simulink model "LMS_cs_old"  (R2023a)
settings: Solver=ode5  StartTime=0.0  StopTime=inf  FixedStep=1/200  RelTol=1e-3
PreLoadFcn:
  | mbxruntime.callbacks.PreLoadFcn(bdroot);
PostLoadFcn:
  | mbxruntime.callbacks.PostLoadFcn(bdroot);
InitFcn:
  | mbxruntime.callbacks.InitFcn(bdroot);
StartFcn:
  | mbxruntime.callbacks.StartFcn(bdroot);
StopFcn:
  | mbxruntime.callbacks.StopFcn(bdroot);
model workspace (MAT data in the model file):
  mbox_table : object (value not decoded)
  model_closed = 0
  sim_status = 0
undefined symbols (not defined in the file or in its folder): DiscIntNeverNeededParam, WheelL0, WheelL1, WheelR0, WheelR1
libraries: simulink x462, simulink_extras x117, PreScanSimulinkLibrary x33, PreScanUsefulBlocks x6, instrumentseriallib x5, simulink_need_slupdate x1
(part 41 of 68)

== system LMS_cs_old/BMW_X5_SUV_8/Dynamics_Simple_3D/Chassis/Bicycle_model_[XYZ] ==
  DeltaWheel_[rad] : Inport
  BrakePressure_[bar] : Inport  Port=2
  DriveTorque_[Nm] : Inport  Port=3
  v0_[ms-1] : Inport  Port=4
  |vx|_[ms-1] : Inport  Port=5
  Fy_rear_[N] : Inport  Port=6
  Fy_front_[N] : Inport  Port=7
  TyreInfo_in : Inport  Port=8
  Bus Creator : BusCreator  Inputs=4
  Fyi --> Fy / Mz : Subsystem
  Goto Tag Visibility2 : GotoTagVisibility  GotoTag=penetrationfrontleft
  Goto Tag Visibility3 : GotoTagVisibility  GotoTag=penetrationfrontright
  Goto Tag Visibility4 : GotoTagVisibility  GotoTag=penetrationrearright
  Goto Tag Visibility5 : GotoTagVisibility  GotoTag=penetrationrearleft
  RoadContact : Subsystem
  Terminator : Terminator
  X_Motion : Subsystem
  Y & Yaw_Motion : Subsystem
  "Z, Pitch_Motion & Roll_Motion" : Subsystem
  Z_Motion unsprung mass : Subsystem
  |vx|_[ms-1]1 : Outport
  vy_[ms-1] : Outport  Port=2
  vz_[ms-1] : Outport  Port=3
  RollAngle_[rad] : Outport  Port=4
  RollRate_[rads-1] : Outport  Port=5
  YawAngle_[rads-1] : Outport  Port=6
  Vx_[ms-1] : Outport  Port=7
  PitchAngle_[rad] : Outport  Port=8
  YawAngle_[rad] : Outport  Port=9
  ax_[ms-2] : Outport  Port=10
  ay_[ms-2] : Outport  Port=11
  z_wheel_[m] : Outport  Port=12
  tag scope: penetrationfrontleft=scoped, penetrationfrontright=scoped, penetrationrearleft=scoped, penetrationrearright=scoped
  wires:
  TyreInfo_in/1 -> RoadContact/1(TyreInfo_in)
  Bus Creator/1 -> z_wheel_[m]/1
  "Z, Pitch_Motion & Roll_Motion"/2(vz_[ms-1]) -> vz_[ms-1]/1  "vz_[ms-1]"
  v0_[ms-1]/1 -> X_Motion/3(v0_[ms-1])  "v0_[ms-1]"
  [slope] -> X_Motion/4(slope_[rad])
  RoadContact/4(depth_RR [m]) -> [penetrationrearright]
  RoadContact/3(depth_RL [m]) -> [penetrationrearleft]
  RoadContact/2(depth_FR [m]) -> [penetrationfrontright]
  RoadContact/1(depth_FL [m]) -> [penetrationfrontleft]
  Y & Yaw_Motion/5(YawAngle_[rad]) -> YawAngle_[rad]/1  "YawAngle_[rad]"
  [az] -> Z_Motion unsprung mass/2(az_[ms-2])
  [FdampRR] -> Z_Motion unsprung mass/10(FdampRR_[N])
  [FdampRL] -> Z_Motion unsprung mass/9(FdampRL_[N])
  [FspringRR] -> Z_Motion unsprung mass/8(FspringRR_[N])
  [FspringRL] -> Z_Motion unsprung mass/7(FspringRL_[N])
  [FdampFR] -> Z_Motion unsprung mass/6(FdampFR_[N])
  [FdampFL] -> Z_Motion unsprung mass/5(FdampFL_[N])
  [FspringFR] -> Z_Motion unsprung mass/4(FspringFR_[N])
  [FspringFL] -> Z_Motion unsprung mass/3(FspringFL_[N])
  [pitch] -> Z_Motion unsprung mass/1(pitch_[rad])
  Z_Motion unsprung mass/4(z_wheelRR_[m]) -> Bus Creator/4, [z_wheelRR]  "z_wheelRR_[m]"
  Z_Motion unsprung mass/3(z_wheelRL_[m]) -> Bus Creator/3, [z_wheelRL]  "z_wheelRL_[m]"
  Z_Motion unsprung mass/2(z_wheelFR_[m]) -> Bus Creator/2, [z_wheelFR]  "z_wheelFR_[m]"
  Z_Motion unsprung mass/1(z_wheelFL_[m]) -> Bus Creator/1, [z_wheelFL]  "z_wheelFL_[m]"
  [z_wheelRR] -> "Z, Pitch_Motion & Roll_Motion"/9(z_wheelRR_[m])
  [z_wheelRL] -> "Z, Pitch_Motion & Roll_Motion"/8(z_wheelRL_[m])
  [z_wheelFR] -> "Z, Pitch_Motion & Roll_Motion"/7(z_wheelFR_[m])
  [z_wheelFL] -> "Z, Pitch_Motion & Roll_Motion"/6(z_wheelFL_[m])
  [pitch] -> "Z, Pitch_Motion & Roll_Motion"/1(pitch_[rad])
  "Z, Pitch_Motion & Roll_Motion"/13(FdampRR_[N]) -> [FdampRR]
  "Z, Pitch_Motion & Roll_Motion"/12(FdampRL_[N]) -> [FdampRL]
  "Z, Pitch_Motion & Roll_Motion"/11(FspringRR_[N]) -> [FspringRR]
  "Z, Pitch_Motion & Roll_Motion"/10(FspringRL_[N]) -> [FspringRL]
  "Z, Pitch_Motion & Roll_Motion"/9(FdampFR_[N]) -> [FdampFR]
  "Z, Pitch_Motion & Roll_Motion"/8(FdampFL_[N]) -> [FdampFL]
  "Z, Pitch_Motion & Roll_Motion"/7(FspringFR_[N]) -> [FspringFR]
  "Z, Pitch_Motion & Roll_Motion"/6(FspringFL_[N]) -> [FspringFL]
  "Z, Pitch_Motion & Roll_Motion"/5(RollRate_[rads-1]) -> RollRate_[rads-1]/1
  "Z, Pitch_Motion & Roll_Motion"/3(az_[ms-2]) -> [az]
  [dYaw] -> X_Motion/6(dYaw_[rads-1])
  [vy] -> X_Motion/5(vy_[ms-1])
  Fyi --> Fy / Mz/1(Fy_[N]) -> Y & Yaw_Motion/2(Fy_[N])  "Fy_[N]"
  Fyi --> Fy / Mz/2(Mz_[Nm]) -> Y & Yaw_Motion/3(Mz_[Nm])  "Mz_[Nm]"
  Y & Yaw_Motion/1(|vx|_[ms-1]1) -> |vx|_[ms-1]1/1  "|vx|_[ms-1]"
  Y & Yaw_Motion/2(vy_[ms-1]) -> [vy], vy_[ms-1]/1  "vy_[ms-1]"
  BrakePressure_[bar]/1 -> X_Motion/2(BrakePressure_[bar])  "BrakePressure_[bar]"
  DriveTorque_[Nm]/1 -> X_Motion/1(DriveTorque_[Nm])  "DriveTorque_[Nm]"
  X_Motion/2(ax_[ms-2]) -> ax_[ms-2]/1, [ax]  "ax_[ms-2]"
  X_Motion/1(vx_[ms-1]) -> Vx_[ms-1]/1, [vx]  "vx_[ms-1]"
  [ax] -> "Z, Pitch_Motion & Roll_Motion"/4(ax)
  DeltaWheel_[rad]/1 -> Fyi --> Fy / Mz/1(DeltaWheel_[rad])
  Fy_front_[N]/1 -> Fyi --> Fy / Mz/2(Fy_f_[N])
  Fy_rear_[N]/1 -> Fyi --> Fy / Mz/3(Fy_r_[N])
  |vx|_[ms-1]/1 -> Y & Yaw_Motion/1(|vx|_[ms-1])
  Y & Yaw_Motion/3(ay_[ms-2]) -> [ay], ay_[ms-2]/1
  [ay] -> "Z, Pitch_Motion & Roll_Motion"/5(ay)
  "Z, Pitch_Motion & Roll_Motion"/4(RollAngle_[rad]) -> RollAngle_[rad]/1
  [dYaw] -> "Z, Pitch_Motion & Roll_Motion"/3(dYaw)
  [vx] -> "Z, Pitch_Motion & Roll_Motion"/2(vx)
  Y & Yaw_Motion/4(dYawAngle_[rads-1]) -> YawAngle_[rads-1]/1, [dYaw]  "dYawAngle_[rads-1]"
  "Z, Pitch_Motion & Roll_Motion"/1(pitchAngle_[rad]) -> [pitch], PitchAngle_[rad]/1  "PitchAngle_[rad]"
  RoadContact/5(z) -> Terminator/1
  RoadContact/6(slope) -> [slope]
  RoadContact/7(banking) -> [banking]
  [banking] -> "Z, Pitch_Motion & Roll_Motion"/10(banking)

== system LMS_cs_old/BMW_X5_SUV_8/Dynamics_Simple_3D/Chassis/FrontTyre ==
  note: relax_on
      | ON: 1
      | OFF: 0
  note: MOTORCYCLE ONLY
  note: VEHICLE + MOTORCYCLE
  note: alpha limiter
      | [-1 ... 1]
  DeltaWheel_[rad] : Inport
  |vx|_[ms-1] : Inport  Port=2
  vy_[ms-1] : Inport  Port=3
  dYawAngle_[rads-1] : Inport  Port=4
  RollAngle_[rad] : Inport  Port=5
  AlphaFront : Subsystem
  Compare To Zero : simulink/Logic and Bit Operations/Compare To Zero  relop===  OutDataTypeStr=boolean  ZeroCross=off
  Configurable Subsystem : Subsystem  BlockChoice=Integrator  mask{ComputationMode=ComputationMode}
      mask prompts: ComputationMode "Computation mode:"
      mask init:
      | SetComputationMode(gcb,ComputationMode);
      settings: AttributesFormatString=%<BlockChoice>  OpenFcn=BringToFront(gcb);  MemberBlocks=Discrete-Time Integrator,Integrator
      settings: TemplateBlock=|
      | PreScanSimulinkLibrary/Configurable Subsystems/integral with reset and limits
      | for slip angle/Configurable
      | Subsystem
  Configurable Subsystem1 : Subsystem  BlockChoice=Integrator  mask{ComputationMode=ComputationMode}
      mask prompts: ComputationMode "Computation mode:"
      mask init:
      | SetComputationMode(gcb,ComputationMode);
      settings: AttributesFormatString=%<BlockChoice>  OpenFcn=BringToFront(gcb);  MemberBlocks=Discrete-Time Integrator,Integrator
      settings: TemplateBlock=|
      | PreScanSimulinkLibrary/Configurable Subsystems/integral with reset/Configurable
      | Subsystem
  Constant : Constant  Value=p.relax_on
  Constant1 : Constant  Value=p.relax_on
  Constant2 : Constant  Value=p.VehMCSwitch
  Data Type Conversion : DataTypeConversion  OutDataTypeStr=double  SaturateOnIntegerOverflow=off  RndMeth=Floor
  If MC : simulink/Logic and Bit Operations/Compare To Constant  relop===  const=2  OutDataTypeStr=uint8  ZeroCross=off
  K_gamma_front : Gain  Gain=p.Kgfront
  Linl : Fcn  Expr=(u(4) - u(5))/p.sigma_front*u(1)
  Linl1 : Fcn  Expr=(u(4) - u(5))/p.sigma_front*u(1)
  Mux1 : Mux  Inputs=3
  Mux2 : Mux  Inputs={3,1,1}
  Mux3 : Mux  Inputs={3,1,1}
  Product : Product  RndMeth=Zero
  Sum : Sum  Inputs=|++  InputSameDT=on  SaturateOnIntegerOverflow=on  OutDataTypeStr=Inherit: Same as first input
  Sum1 : Sum  Inputs=|++
  Switch : Switch  Threshold=0.5
  Switch1 : Switch  Threshold=0.5
  alg.loop : Memory
  due to sign convention : Gain  Gain=-1  SaturateOnIntegerOverflow=on  OutDataTypeStr=Inherit: Same as input  ParamDataTypeStr=Inherit: Same as input
  front_tyre : Gain  Gain=p.Kfront
  FyFront_[N] : Outport
  wires:
  Sum/1 -> Mux2/2, Switch/3  "AlphaStatFront_[rad]"
  Switch/1 -> front_tyre/1  "AlphaFront_[rad]"
  Constant/1 -> Switch/2
  Sum1/1 -> FyFront_[N]/1  "FyFront_[N]"
  Mux2/1 -> Linl/1
  Linl/1 -> Configurable Subsystem/1(In1)
  Configurable Subsystem/1(Out1) -> Mux2/3, Switch/1  "AlphaRelaxFront_[rad]"
  AlphaFront/1(Alpha) -> Sum/1
  Mux1/1 -> AlphaFront/1(In), Mux2/1, Mux3/1
  |vx|_[ms-1]/1 -> Mux1/1, Compare To Zero/1
  vy_[ms-1]/1 -> Mux1/2
  dYawAngle_[rads-1]/1 -> Mux1/3
  alg.loop/1 -> Switch1/3
  Configurable Subsystem1/1(Out1) -> Mux3/3, Switch1/1  "GammaRelaxFront_[rad]"
  Linl1/1 -> Configurable Subsystem1/1(In1)
  Mux3/1 -> Linl1/1
  Constant1/1 -> Switch1/2
  due to sign convention/1 -> alg.loop/1, Mux3/2  "GammaStatFront_[rad]"
  RollAngle_[rad]/1 -> due to sign convention/1
  front_tyre/1 -> Sum1/1
  Constant2/1 -> If MC/1
  If MC/1 -> Data Type Conversion/1
  K_gamma_front/1 -> Product/1
  Product/1 -> Sum1/2
  Data Type Conversion/1 -> Product/2
  Compare To Zero/1 -> [reset]
  [reset] -> Configurable Subsystem/2(In2)
  [reset] -> Configurable Subsystem1/2(In2)
  DeltaWheel_[rad]/1 -> Sum/2  "DeltaWheel_[rad]"
  Switch1/1 -> K_gamma_front/1  "GammaFront_[rad]"

== system LMS_cs_old/BMW_X5_SUV_8/Dynamics_Simple_3D/Chassis/Power Assisted Steering ==
  note: MOTORCYCLE
  note: VEHICLE
  note: Reverse steering direction for negative velocities
  Vx_[ms-1] : Inport
  Delta_in_[deg] : Inport  Port=2
  Constant : Constant
  Constant1 : Constant  Value=p.VehMCSwitch
  Lookup Table : Lookup  InputValues=[0 35 45 100]  Table=[1 1 0.2 0.2]  SaturateOnIntegerOverflow=off
  Multiport Switch : MultiPortSwitch  Inputs=2  SaturateOnIntegerOverflow=off  InputSameDT=off
  Product : Product  Inputs=3  RndMeth=Zero
  Sign : Signum
  Delta_out_[deg] : Outport
  wires:
  Vx_[ms-1]/1 -> Lookup Table/1, Sign/1
  Delta_in_[deg]/1 -> Product/3
  Constant1/1 -> Multiport Switch/1
  Constant/1 -> Multiport Switch/3
  Lookup Table/1 -> Multiport Switch/2
  Multiport Switch/1 -> Product/2
  Product/1 -> Delta_out_[deg]/1
  Sign/1 -> Product/1

== system LMS_cs_old/BMW_X5_SUV_8/Dynamics_Simple_3D/Chassis/RearTyre ==
  note: relax_on
      | ON: 1
      | OFF: 0
  note: MOTORCYCLE ONLY
  note: VEHICLE + MOTORCYCLE
  note: alpha limiter
      | [-1 ... 1]
  |vx|_[ms-1] : Inport
  vy_[ms-1] : Inport  Port=2
  dpsi_[rads-1] : Inport  Port=3
  RollAngle_[rad] : Inport  Port=4
  AlphaRear : Subsystem
  Compare To Zero : simulink/Logic and Bit Operations/Compare To Zero  relop===  OutDataTypeStr=boolean  ZeroCross=off
  Configurable Subsystem : Subsystem  BlockChoice=Integrator  mask{ComputationMode=ComputationMode}
      mask prompts: ComputationMode "Computation mode:"
      mask init:
      | SetComputationMode(gcb,ComputationMode);
      settings: AttributesFormatString=%<BlockChoice>  OpenFcn=BringToFront(gcb);  MemberBlocks=Discrete-Time Integrator,Integrator
      settings: TemplateBlock=|
      | PreScanSimulinkLibrary/Configurable Subsystems/integral with reset and limits
      | for slip angle/Configurable
      | Subsystem
  Configurable Subsystem1 : Subsystem  BlockChoice=Integrator  mask{ComputationMode=ComputationMode}
      mask prompts: ComputationMode "Computation mode:"
      mask init:
      | SetComputationMode(gcb,ComputationMode);
      settings: AttributesFormatString=%<BlockChoice>  OpenFcn=BringToFront(gcb);  MemberBlocks=Discrete-Time Integrator,Integrator
      settings: TemplateBlock=|
      | PreScanSimulinkLibrary/Configurable Subsystems/integral with reset/Configurable
      | Subsystem
  Constant1 : Constant  Value=p.relax_on
  Constant2 : Constant  Value=p.relax_on
  Constant3 : Constant  Value=p.VehMCSwitch
  Data Type Conversion : DataTypeConversion  OutDataTypeStr=double  SaturateOnIntegerOverflow=off  RndMeth=Floor
  If MC : simulink/Logic and Bit Operations/Compare To Constant  relop===  const=2  OutDataTypeStr=uint8  ZeroCross=off
  K_gamma_rear : Gain  Gain=p.Kgrear
  Linl : Fcn  Expr=(u(4) - u(5))/p.sigma_rear*u(1)
  Linl1 : Fcn  Expr=(u(4) - u(5))/p.sigma_rear*u(1)
  Mux1 : Mux  Inputs=3
  Mux2 : Mux  Inputs={3,1,1}
  Mux3 : Mux  Inputs={3,1,1}
  Product : Product  RndMeth=Zero
  Sum1 : Sum  Inputs=|++
  Switch1 : Switch  Threshold=0.5
  Switch2 : Switch  Threshold=0.5
  alg.loop : Memory
  due to sign convention : Gain  Gain=-1  SaturateOnIntegerOverflow=on  OutDataTypeStr=Inherit: Same as input  ParamDataTypeStr=Inherit: Same as input
  rear_tyre : Gain  Gain=p.Krear
  FyRear_[N] : Outport
  wires:
  AlphaRear/1(Alpha) -> Switch1/3, Mux2/2  "AlphaStatRear_[rad]"
  Switch1/1 -> rear_tyre/1  "AlphaRear_[rad]"
  Constant1/1 -> Switch1/2
  Sum1/1 -> FyRear_[N]/1  "FyRear_[N]"
  Mux2/1 -> Linl/1
  Linl/1 -> Configurable Subsystem/1(In1)
  Configurable Subsystem/1(Out1) -> Mux2/3, Switch1/1  "AlphaRelaxRear_[rad]"
  Mux1/1 -> AlphaRear/1(In), Mux2/1, Mux3/1
  |vx|_[ms-1]/1 -> Mux1/1, Compare To Zero/1
  vy_[ms-1]/1 -> Mux1/2
  dpsi_[rads-1]/1 -> Mux1/3
  alg.loop/1 -> Switch2/3
  Configurable Subsystem1/1(Out1) -> Mux3/3, Switch2/1  "GammaRelaxRear_[rad]"
  Linl1/1 -> Configurable Subsystem1/1(In1)
  Mux3/1 -> Linl1/1
  Constant2/1 -> Switch2/2
  due to sign convention/1 -> alg.loop/1, Mux3/2  "GammaStatRear_[rad]"
  RollAngle_[rad]/1 -> due to sign convention/1
  Constant3/1 -> If MC/1
  If MC/1 -> Data Type Conversion/1
  Product/1 -> Sum1/2
  Data Type Conversion/1 -> Product/2
  K_gamma_rear/1 -> Product/1
  rear_tyre/1 -> Sum1/1
  Compare To Zero/1 -> [reset]
  [reset] -> Configurable Subsystem/2(In2)
  [reset] -> Configurable Subsystem1/2(In2)
  Switch2/1 -> K_gamma_rear/1  "GammaFront_[rad]"

== system LMS_cs_old/BMW_X5_SUV_8/Dynamics_Simple_3D/Engine/Configurable Subsystem ==
  In1 : Inport
  Rate Limiter : TransferFcn  Denominator=[0.1 1]
  Out1 : Outport
  wires:
  In1/1 -> Rate Limiter/1
  Rate Limiter/1 -> Out1/1

== system LMS_cs_old/BMW_X5_SUV_8/Dynamics_Simple_3D/Engine/Configurable Subsystem1 ==
  In1 : Inport
  Integrator : Integrator  InitialCondition=p.rot_ini  LimitOutput=on  UpperSaturationLimit=p.rot_upp  LowerSaturationLimit=p.rot_low
  Out1 : Outport
  wires:
  In1/1 -> Integrator/1
  Integrator/1 -> Out1/1

== system LMS_cs_old/BMW_X5_SUV_8/Dynamics_Simple_3D/Gear: Auto Manual/If Action Subsystem ==
  In1 : Inport
  Action Port : ActionPort  PropagateVarSize=During execution  ActionPortLabel=if(u1 == 0)
  Out1 : Outport
  wires:
  In1/1 -> Out1/1

== system LMS_cs_old/BMW_X5_SUV_8/Dynamics_Simple_3D/Gear: Auto Manual/If Action Subsystem1 ==
  In1 : Inport
  Action Port : ActionPort  PropagateVarSize=During execution  ActionPortLabel=else
  Out1 : Outport
  wires:
  In1/1 -> Out1/1

== system LMS_cs_old/BMW_X5_SUV_8/Dynamics_Simple_3D/ShiftLogic/Detect Increase ==
  GearNr_[-] : Inport
  In2 : Inport  Port=2
  Constant : Constant
  Data Type Conversion : DataTypeConversion  OutDataTypeStr=double  SaturateOnIntegerOverflow=off  RndMeth=Floor
  Data Type Conversion1 : DataTypeConversion  OutDataTypeStr=double  SaturateOnIntegerOverflow=off  RndMeth=Floor
  Detect Increase : simulink/Logic and Bit Operations/Detect Increase  vinit=1  OutDataTypeStr=uint8
  If : If  NumInputs=2  IfExpression="u1==1 &  u2==1"
  If V0 higher of the from 2->3 shifting velocity : Subsystem  TreatAsAtomicUnit=on
  Merge : Merge
  Other : Subsystem  TreatAsAtomicUnit=on
  Out1 : Outport
  wires:
  In2/1 -> Other/1(In1), Data Type Conversion1/1
  GearNr_[-]/1 -> Detect Increase/1
  Constant/1 -> If V0 higher of the from 2->3 shifting velocity/1(In1)
  Data Type Conversion/1 -> If/1
  Data Type Conversion1/1 -> If/2
  If/1 -> If V0 higher of the from 2->3 shifting velocity/Action
  Merge/1 -> Out1/1
  Detect Increase/1 -> Data Type Conversion/1
  Other/1(Out1) -> Merge/2
  If V0 higher of the from 2->3 shifting velocity/1(Out1) -> Merge/1
  If/2 -> Other/Action

== system LMS_cs_old/BMW_X5_SUV_8/Dynamics_Simple_3D/ShiftLogic/If Action Neutral ==
  In1 : Inport
  Action Port : ActionPort  InitializeStates=reset  PropagateVarSize=During execution  ActionPortLabel=if(u1 == 0)
  Out1 : Outport
  wires:
  In1/1 -> Out1/1

== system LMS_cs_old/BMW_X5_SUV_8/Dynamics_Simple_3D/ShiftLogic/If Action Normal ==
  In1 : Inport
  Action Port : ActionPort  InitializeStates=reset  PropagateVarSize=During execution  ActionPortLabel=else
  Out1 : Outport
  wires:
  In1/1 -> Out1/1

== system LMS_cs_old/BMW_X5_SUV_8/Dynamics_Simple_3D/ShiftLogic/If Action Reverse ==
  In1 : Inport
  Action Port : ActionPort  InitializeStates=reset  PropagateVarSize=During execution  ActionPortLabel=elseif(u1 < 0)
  Out1 : Outport
  wires:
  In1/1 -> Out1/1

== system LMS_cs_old/BMW_X5_SUV_8/Dynamics_Simple_3D/Transmission/Torque_Converter ==
  note: <= 0
  note: > 0
  note: To compensate for no hydraulic connection when in neutral gear
  nEngine_[rpm] : Inport
  nTransmission_[rpm] : Inport  Port=2
  Gear nr : Inport  Port=3
  Compare To Constant : simulink/Logic and Bit Operations/Compare To Constant  relop=<=  const=1  OutDataTypeStr=uint8  ZeroCross=off
  Compare To Zero : simulink/Logic and Bit Operations/Compare To Zero  relop=~=  OutDataTypeStr=uint8  ZeroCross=off
  Constant : Constant  Value=1/50
  Constant1 : Constant
  Constant2 : Constant
  Drag : Gain  Gain=-1
  FactorK : Lookup  InputValues=p.speedratio  Table=p.Kfactor*p.Kcorr
  Impeller : Fcn  Expr=u^2
  Product : Product  RndMeth=Zero
  Product1 : Product  RndMeth=Zero
  Quotient : Product  Inputs=*/  InputSameDT=on  SaturateOnIntegerOverflow=on  OutDataTypeStr=Inherit: Same as first input
  SpeedRatio : Product  Inputs=*/  InputSameDT=on  SaturateOnIntegerOverflow=on  OutDataTypeStr=Inherit: Same as first input
  Sum : Sum  Inputs=|+-
  Switch : Switch  Criteria=u2 ~= 0  Threshold=0.5  SaturateOnIntegerOverflow=off  InputSameDT=off
  Switch1 : Switch  Criteria=u2 ~= 0  SaturateOnIntegerOverflow=off  InputSameDT=off
  TorqueRatio : Lookup  InputValues=[p.speedratio 1]  Table=[p.Torqueratio 0]
  Turbine : Product  InputSameDT=on  SaturateOnIntegerOverflow=on  OutDataTypeStr=Inherit: Same as first input
  rpm2rads-1 : Gain  Gain=2*pi/60
  ImpellerTorque_[Nm] : Outport  InitialOutput=0
  TurbineTorque_[Nm] : Outport  Port=2  InitialOutput=0
  wires:
  rpm2rads-1/1 -> Quotient/1
  Turbine/1 -> Switch1/1
  TorqueRatio/1 -> Turbine/2
  Compare To Constant/1 -> Switch1/2
  Constant2/1 -> Sum/2
  Sum/1 -> Drag/1
  Drag/1 -> Switch1/3
  Product1/1 -> TurbineTorque_[Nm]/1
  Switch1/1 -> Product1/2
  Compare To Zero/1 -> Switch/2
  Gear nr/1 -> Compare To Zero/1
  Constant1/1 -> Switch/1
  Constant/1 -> Switch/3
  Switch/1 -> Product1/1, Product/1
  Product/1 -> ImpellerTorque_[Nm]/1
  Quotient/1 -> Impeller/1
  FactorK/1 -> Quotient/2
  SpeedRatio/1 -> FactorK/1, Sum/1, Compare To Constant/1, TorqueRatio/1
  Impeller/1 -> Turbine/1, Product/2
  nEngine_[rpm]/1 -> SpeedRatio/2, rpm2rads-1/1
  nTransmission_[rpm]/1 -> SpeedRatio/1

== system LMS_cs_old/BMW_X5_SUV_8/Dynamics_Simple_3D/Transmission/Transmission_Ratio ==
  tTransmissionIn_[Nm] : Inport
  GearNr_[-] : Inport  Port=2
  nTransmissionOut_[rpm] : Inport  Port=3
  Ensure positive TransmissionRPM : Abs  SaturateOnIntegerOverflow=off
  If : If  IfExpression=u1 == 0  ElseIfExpressions=u1 == -1
  If Action Neutral : Subsystem  TreatAsAtomicUnit=on
  If Action Normal : Subsystem  TreatAsAtomicUnit=on
  If Action Reverse : Subsystem  TreatAsAtomicUnit=on
  Merge : Merge  Inputs=3
  OutputTorque = 0 : Constant  Value=0
  Product : Product  InputSameDT=on  SaturateOnIntegerOverflow=on  OutDataTypeStr=Inherit: Same as first input
  Product1 : Product  InputSameDT=on  SaturateOnIntegerOverflow=on  OutDataTypeStr=Inherit: Same as first input
  Transmission Gear ratios : Lookup  InputValues=p.tr_in  Table=p.tr_out
  tTransmissionOut_[Nm] : Outport  InitialOutput=0
  nTransmissionIn_[rpm] : Outport  Port=2  InitialOutput=0
  wires:
  Ensure positive TransmissionRPM/1 -> nTransmissionIn_[rpm]/1
  tTransmissionIn_[Nm]/1 -> Product/1
  nTransmissionOut_[rpm]/1 -> Product1/2
  Transmission Gear ratios/1 -> Product1/1, Product/2
  OutputTorque = 0/1 -> If Action Neutral/1(In1)
  Product/1 -> If Action Normal/1(In1), If Action Reverse/1(In1)
  Merge/1 -> tTransmissionOut_[Nm]/1
  Product1/1 -> Ensure positive TransmissionRPM/1
  If Action Neutral/1(Out1) -> Merge/1
  If/1 -> If Action Neutral/Action
  If Action Reverse/1(Out1) -> Merge/2
  If Action Normal/1(Out1) -> Merge/3
  If/2 -> If Action Reverse/Action
  If/3 -> If Action Normal/Action
  GearNr_[-]/1 -> If/1, Transmission Gear ratios/1

== system LMS_cs_old/BMW_X5_SUV_8/PreScan_Contact_Sensor/Tire Collision Demux/Contact Point Bus Creator ==
  demux in : Inport
  Bus Creator : BusCreator  Inputs=3
  Bus Creator1 : BusCreator  Inputs=3
  Bus Creator2 : BusCreator  Inputs=3
  Demux : Demux  Outputs=3
  Demux5 : Demux  Outputs=[3 3 1]
  Demux6 : Demux  Outputs=3
  bus out : Outport
  wires:
  Demux/1 -> Bus Creator/1  "x"
  Demux/2 -> Bus Creator/2  "y"
  Demux/3 -> Bus Creator/3  "z"
  Demux6/1 -> Bus Creator1/1  "x"
  Demux6/2 -> Bus Creator1/2  "y"
  Demux6/3 -> Bus Creator1/3  "z"
  demux in/1 -> Demux5/1
  Demux5/3 -> Bus Creator2/3  "penetrationdepth"
  Bus Creator2/1 -> bus out/1
  Demux5/1 -> Demux/1
  Demux5/2 -> Demux6/1
  Bus Creator/1 -> Bus Creator2/1  "normal"
  Bus Creator1/1 -> Bus Creator2/2  "position"

== system LMS_cs_old/BMW_X5_SUV_8/PreScan_Contact_Sensor/Tire Collision Demux/Contact Point Bus Creator1 ==
  demux in : Inport
  Bus Creator : BusCreator  Inputs=3
  Bus Creator1 : BusCreator  Inputs=3
  Bus Creator2 : BusCreator  Inputs=3
  Demux : Demux  Outputs=3
  Demux5 : Demux  Outputs=[3 3 1]
  Demux6 : Demux  Outputs=3
  bus out : Outport
  wires:
  Demux/1 -> Bus Creator/1  "x"
  Demux/2 -> Bus Creator/2  "y"
  Demux/3 -> Bus Creator/3  "z"
  Demux6/1 -> Bus Creator1/1  "x"
  Demux6/2 -> Bus Creator1/2  "y"
  Demux6/3 -> Bus Creator1/3  "z"
  demux in/1 -> Demux5/1
  Demux5/3 -> Bus Creator2/3  "penetrationdepth"
  Bus Creator2/1 -> bus out/1
  Demux5/1 -> Demux/1
  Demux5/2 -> Demux6/1
  Bus Creator/1 -> Bus Creator2/1  "normal"
  Bus Creator1/1 -> Bus Creator2/2  "position"

== system LMS_cs_old/BMW_X5_SUV_8/PreScan_Contact_Sensor/Tire Collision Demux/Contact Point Bus Creator2 ==
  demux in : Inport
  Bus Creator : BusCreator  Inputs=3
  Bus Creator1 : BusCreator  Inputs=3
  Bus Creator2 : BusCreator  Inputs=3
  Demux : Demux  Outputs=3
  Demux5 : Demux  Outputs=[3 3 1]
  Demux6 : Demux  Outputs=3
  bus out : Outport
  wires:
  Demux/1 -> Bus Creator/1  "x"
  Demux/2 -> Bus Creator/2  "y"
  Demux/3 -> Bus Creator/3  "z"
  Demux6/1 -> Bus Creator1/1  "x"
  Demux6/2 -> Bus Creator1/2  "y"
  Demux6/3 -> Bus Creator1/3  "z"
  demux in/1 -> Demux5/1
  Demux5/3 -> Bus Creator2/3  "penetrationdepth"
  Bus Creator2/1 -> bus out/1
  Demux5/1 -> Demux/1
  Demux5/2 -> Demux6/1
  Bus Creator/1 -> Bus Creator2/1  "normal"
  Bus Creator1/1 -> Bus Creator2/2  "position"

== system LMS_cs_old/BMW_X5_SUV_8/PreScan_Contact_Sensor/Tire Collision Demux/Contact Point Bus Creator3 ==
  demux in : Inport
  Bus Creator : BusCreator  Inputs=3
  Bus Creator1 : BusCreator  Inputs=3
  Bus Creator2 : BusCreator  Inputs=3
  Demux : Demux  Outputs=3
  Demux5 : Demux  Outputs=[3 3 1]
  Demux6 : Demux  Outputs=3
  bus out : Outport
  wires:
  Demux/1 -> Bus Creator/1  "x"
  Demux/2 -> Bus Creator/2  "y"
  Demux/3 -> Bus Creator/3  "z"
  Demux6/1 -> Bus Creator1/1  "x"
  Demux6/2 -> Bus Creator1/2  "y"
  Demux6/3 -> Bus Creator1/3  "z"
  demux in/1 -> Demux5/1
  Demux5/3 -> Bus Creator2/3  "penetrationdepth"
  Bus Creator2/1 -> bus out/1
  Demux5/1 -> Demux/1
  Demux5/2 -> Demux6/1
  Bus Creator/1 -> Bus Creator2/1  "normal"
  Bus Creator1/1 -> Bus Creator2/2  "position"

== system LMS_cs_old/BMW_X5_SUV_8/PreScan_Contact_Sensor/Tire Collision Demux1/Contact Point Bus Creator ==
  demux in : Inport
  Bus Creator : BusCreator  Inputs=3
  Bus Creator1 : BusCreator  Inputs=3
  Bus Creator2 : BusCreator  Inputs=3
  Demux : Demux  Outputs=3
  Demux5 : Demux  Outputs=[3 3 1]
  Demux6 : Demux  Outputs=3
  bus out : Outport
  wires:
  Demux/1 -> Bus Creator/1  "x"
  Demux/2 -> Bus Creator/2  "y"
  Demux/3 -> Bus Creator/3  "z"
  Demux6/1 -> Bus Creator1/1  "x"
  Demux6/2 -> Bus Creator1/2  "y"
  Demux6/3 -> Bus Creator1/3  "z"
  demux in/1 -> Demux5/1
  Demux5/3 -> Bus Creator2/3  "penetrationdepth"
  Bus Creator2/1 -> bus out/1
  Demux5/1 -> Demux/1
  Demux5/2 -> Demux6/1
  Bus Creator/1 -> Bus Creator2/1  "normal"
  Bus Creator1/1 -> Bus Creator2/2  "position"

== system LMS_cs_old/BMW_X5_SUV_8/PreScan_Contact_Sensor/Tire Collision Demux1/Contact Point Bus Creator1 ==
  demux in : Inport
  Bus Creator : BusCreator  Inputs=3
  Bus Creator1 : BusCreator  Inputs=3
  Bus Creator2 : BusCreator  Inputs=3
  Demux : Demux  Outputs=3
  Demux5 : Demux  Outputs=[3 3 1]
  Demux6 : Demux  Outputs=3
  bus out : Outport
  wires:
  Demux/1 -> Bus Creator/1  "x"
  Demux/2 -> Bus Creator/2  "y"
  Demux/3 -> Bus Creator/3  "z"
  Demux6/1 -> Bus Creator1/1  "x"
  Demux6/2 -> Bus Creator1/2  "y"
  Demux6/3 -> Bus Creator1/3  "z"
  demux in/1 -> Demux5/1
  Demux5/3 -> Bus Creator2/3  "penetrationdepth"
  Bus Creator2/1 -> bus out/1
  Demux5/1 -> Demux/1
  Demux5/2 -> Demux6/1
  Bus Creator/1 -> Bus Creator2/1  "normal"
  Bus Creator1/1 -> Bus Creator2/2  "position"

== system LMS_cs_old/BMW_X5_SUV_8/PreScan_Contact_Sensor/Tire Collision Demux1/Contact Point Bus Creator2 ==
  demux in : Inport
  Bus Creator : BusCreator  Inputs=3
  Bus Creator1 : BusCreator  Inputs=3
  Bus Creator2 : BusCreator  Inputs=3
  Demux : Demux  Outputs=3
  Demux5 : Demux  Outputs=[3 3 1]
  Demux6 : Demux  Outputs=3
  bus out : Outport
  wires:
  Demux/1 -> Bus Creator/1  "x"
  Demux/2 -> Bus Creator/2  "y"
  Demux/3 -> Bus Creator/3  "z"
  Demux6/1 -> Bus Creator1/1  "x"
  Demux6/2 -> Bus Creator1/2  "y"
  Demux6/3 -> Bus Creator1/3  "z"
  demux in/1 -> Demux5/1
  Demux5/3 -> Bus Creator2/3  "penetrationdepth"
  Bus Creator2/1 -> bus out/1
  Demux5/1 -> Demux/1
  Demux5/2 -> Demux6/1
  Bus Creator/1 -> Bus Creator2/1  "normal"
  Bus Creator1/1 -> Bus Creator2/2  "position"

== system LMS_cs_old/BMW_X5_SUV_8/PreScan_Contact_Sensor/Tire Collision Demux1/Contact Point Bus Creator3 ==
  demux in : Inport
  Bus Creator : BusCreator  Inputs=3
  Bus Creator1 : BusCreator  Inputs=3
  Bus Creator2 : BusCreator  Inputs=3
  Demux : Demux  Outputs=3
  Demux5 : Demux  Outputs=[3 3 1]
  Demux6 : Demux  Outputs=3
  bus out : Outport
  wires:
  Demux/1 -> Bus Creator/1  "x"
  Demux/2 -> Bus Creator/2  "y"
  Demux/3 -> Bus Creator/3  "z"
  Demux6/1 -> Bus Creator1/1  "x"
  Demux6/2 -> Bus Creator1/2  "y"
  Demux6/3 -> Bus Creator1/3  "z"
  demux in/1 -> Demux5/1
  Demux5/3 -> Bus Creator2/3  "penetrationdepth"
  Bus Creator2/1 -> bus out/1
  Demux5/1 -> Demux/1
  Demux5/2 -> Demux6/1
  Bus Creator/1 -> Bus Creator2/1  "normal"
  Bus Creator1/1 -> Bus Creator2/2  "position"

== system LMS_cs_old/BMW_X5_SUV_8/PreScan_Contact_Sensor/Tire Collision Demux2/Contact Point Bus Creator ==
  demux in : Inport
  Bus Creator : BusCreator  Inputs=3
  Bus Creator1 : BusCreator  Inputs=3
  Bus Creator2 : BusCreator  Inputs=3
  Demux : Demux  Outputs=3
  Demux5 : Demux  Outputs=[3 3 1]
  Demux6 : Demux  Outputs=3
  bus out : Outport
  wires:
  Demux/1 -> Bus Creator/1  "x"
  Demux/2 -> Bus Creator/2  "y"
  Demux/3 -> Bus Creator/3  "z"
  Demux6/1 -> Bus Creator1/1  "x"
  Demux6/2 -> Bus Creator1/2  "y"
  Demux6/3 -> Bus Creator1/3  "z"
  demux in/1 -> Demux5/1
  Demux5/3 -> Bus Creator2/3  "penetrationdepth"
  Bus Creator2/1 -> bus out/1
  Demux5/1 -> Demux/1
  Demux5/2 -> Demux6/1
  Bus Creator/1 -> Bus Creator2/1  "normal"
  Bus Creator1/1 -> Bus Creator2/2  "position"

== system LMS_cs_old/BMW_X5_SUV_8/PreScan_Contact_Sensor/Tire Collision Demux2/Contact Point Bus Creator1 ==
  demux in : Inport
  Bus Creator : BusCreator  Inputs=3
  Bus Creator1 : BusCreator  Inputs=3
  Bus Creator2 : BusCreator  Inputs=3
  Demux : Demux  Outputs=3
  Demux5 : Demux  Outputs=[3 3 1]
  Demux6 : Demux  Outputs=3
  bus out : Outport
  wires:
  Demux/1 -> Bus Creator/1  "x"
  Demux/2 -> Bus Creator/2  "y"
  Demux/3 -> Bus Creator/3  "z"
  Demux6/1 -> Bus Creator1/1  "x"
  Demux6/2 -> Bus Creator1/2  "y"
  Demux6/3 -> Bus Creator1/3  "z"
  demux in/1 -> Demux5/1
  Demux5/3 -> Bus Creator2/3  "penetrationdepth"
  Bus Creator2/1 -> bus out/1
  Demux5/1 -> Demux/1
  Demux5/2 -> Demux6/1
  Bus Creator/1 -> Bus Creator2/1  "normal"
  Bus Creator1/1 -> Bus Creator2/2  "position"

== system LMS_cs_old/BMW_X5_SUV_8/PreScan_Contact_Sensor/Tire Collision Demux2/Contact Point Bus Creator2 ==
  demux in : Inport
  Bus Creator : BusCreator  Inputs=3
  Bus Creator1 : BusCreator  Inputs=3
  Bus Creator2 : BusCreator  Inputs=3
  Demux : Demux  Outputs=3
  Demux5 : Demux  Outputs=[3 3 1]
  Demux6 : Demux  Outputs=3
  bus out : Outport
  wires:
  Demux/1 -> Bus Creator/1  "x"
  Demux/2 -> Bus Creator/2  "y"
  Demux/3 -> Bus Creator/3  "z"
  Demux6/1 -> Bus Creator1/1  "x"
  Demux6/2 -> Bus Creator1/2  "y"
  Demux6/3 -> Bus Creator1/3  "z"
  demux in/1 -> Demux5/1
  Demux5/3 -> Bus Creator2/3  "penetrationdepth"
  Bus Creator2/1 -> bus out/1
  Demux5/1 -> Demux/1
  Demux5/2 -> Demux6/1
  Bus Creator/1 -> Bus Creator2/1  "normal"
  Bus Creator1/1 -> Bus Creator2/2  "position"

== system LMS_cs_old/BMW_X5_SUV_8/PreScan_Contact_Sensor/Tire Collision Demux2/Contact Point Bus Creator3 ==
  demux in : Inport
  Bus Creator : BusCreator  Inputs=3
  Bus Creator1 : BusCreator  Inputs=3
  Bus Creator2 : BusCreator  Inputs=3
  Demux : Demux  Outputs=3
  Demux5 : Demux  Outputs=[3 3 1]
  Demux6 : Demux  Outputs=3
  bus out : Outport
  wires:
  Demux/1 -> Bus Creator/1  "x"
  Demux/2 -> Bus Creator/2  "y"
  Demux/3 -> Bus Creator/3  "z"
  Demux6/1 -> Bus Creator1/1  "x"
  Demux6/2 -> Bus Creator1/2  "y"
  Demux6/3 -> Bus Creator1/3  "z"
  demux in/1 -> Demux5/1
  Demux5/3 -> Bus Creator2/3  "penetrationdepth"
  Bus Creator2/1 -> bus out/1
  Demux5/1 -> Demux/1
  Demux5/2 -> Demux6/1
  Bus Creator/1 -> Bus Creator2/1  "normal"
  Bus Creator1/1 -> Bus Creator2/2  "position"

== system LMS_cs_old/BMW_X5_SUV_8/PreScan_Contact_Sensor/Tire Collision Demux3/Contact Point Bus Creator ==
  demux in : Inport
  Bus Creator : BusCreator  Inputs=3
  Bus Creator1 : BusCreator  Inputs=3
  Bus Creator2 : BusCreator  Inputs=3
  Demux : Demux  Outputs=3
  Demux5 : Demux  Outputs=[3 3 1]
  Demux6 : Demux  Outputs=3
  bus out : Outport
  wires:
  Demux/1 -> Bus Creator/1  "x"
  Demux/2 -> Bus Creator/2  "y"
  Demux/3 -> Bus Creator/3  "z"
  Demux6/1 -> Bus Creator1/1  "x"
  Demux6/2 -> Bus Creator1/2  "y"
  Demux6/3 -> Bus Creator1/3  "z"
  demux in/1 -> Demux5/1
  Demux5/3 -> Bus Creator2/3  "penetrationdepth"
  Bus Creator2/1 -> bus out/1
  Demux5/1 -> Demux/1
  Demux5/2 -> Demux6/1
  Bus Creator/1 -> Bus Creator2/1  "normal"
  Bus Creator1/1 -> Bus Creator2/2  "position"

== system LMS_cs_old/BMW_X5_SUV_8/PreScan_Contact_Sensor/Tire Collision Demux3/Contact Point Bus Creator1 ==
  demux in : Inport
  Bus Creator : BusCreator  Inputs=3
  Bus Creator1 : BusCreator  Inputs=3
  Bus Creator2 : BusCreator  Inputs=3
  Demux : Demux  Outputs=3
  Demux5 : Demux  Outputs=[3 3 1]
  Demux6 : Demux  Outputs=3
  bus out : Outport
  wires:
  Demux/1 -> Bus Creator/1  "x"
  Demux/2 -> Bus Creator/2  "y"
  Demux/3 -> Bus Creator/3  "z"
  Demux6/1 -> Bus Creator1/1  "x"
  Demux6/2 -> Bus Creator1/2  "y"
  Demux6/3 -> Bus Creator1/3  "z"
  demux in/1 -> Demux5/1
  Demux5/3 -> Bus Creator2/3  "penetrationdepth"
  Bus Creator2/1 -> bus out/1
  Demux5/1 -> Demux/1
  Demux5/2 -> Demux6/1
  Bus Creator/1 -> Bus Creator2/1  "normal"
  Bus Creator1/1 -> Bus Creator2/2  "position"

== system LMS_cs_old/BMW_X5_SUV_8/PreScan_Contact_Sensor/Tire Collision Demux3/Contact Point Bus Creator2 ==
  demux in : Inport
  Bus Creator : BusCreator  Inputs=3
  Bus Creator1 : BusCreator  Inputs=3
  Bus Creator2 : BusCreator  Inputs=3
  Demux : Demux  Outputs=3
  Demux5 : Demux  Outputs=[3 3 1]
  Demux6 : Demux  Outputs=3
  bus out : Outport
  wires:
  Demux/1 -> Bus Creator/1  "x"
  Demux/2 -> Bus Creator/2  "y"
  Demux/3 -> Bus Creator/3  "z"
  Demux6/1 -> Bus Creator1/1  "x"
  Demux6/2 -> Bus Creator1/2  "y"
  Demux6/3 -> Bus Creator1/3  "z"
  demux in/1 -> Demux5/1
  Demux5/3 -> Bus Creator2/3  "penetrationdepth"
  Bus Creator2/1 -> bus out/1
  Demux5/1 -> Demux/1
  Demux5/2 -> Demux6/1
  Bus Creator/1 -> Bus Creator2/1  "normal"
  Bus Creator1/1 -> Bus Creator2/2  "position"

== system LMS_cs_old/BMW_X5_SUV_8/PreScan_Contact_Sensor/Tire Collision Demux3/Contact Point Bus Creator3 ==
  demux in : Inport
  Bus Creator : BusCreator  Inputs=3
  Bus Creator1 : BusCreator  Inputs=3
  Bus Creator2 : BusCreator  Inputs=3
  Demux : Demux  Outputs=3
  Demux5 : Demux  Outputs=[3 3 1]
  Demux6 : Demux  Outputs=3
  bus out : Outport
  wires:
  Demux/1 -> Bus Creator/1  "x"
  Demux/2 -> Bus Creator/2  "y"
  Demux/3 -> Bus Creator/3  "z"
  Demux6/1 -> Bus Creator1/1  "x"
  Demux6/2 -> Bus Creator1/2  "y"
  Demux6/3 -> Bus Creator1/3  "z"
  demux in/1 -> Demux5/1
  Demux5/3 -> Bus Creator2/3  "penetrationdepth"
  Bus Creator2/1 -> bus out/1
  Demux5/1 -> Demux/1
  Demux5/2 -> Demux6/1
  Bus Creator/1 -> Bus Creator2/1  "normal"
  Bus Creator1/1 -> Bus Creator2/2  "position"

== system LMS_cs_old/BMW_X5_SUV_8/PreScan_Contact_Sensor/Vehicle Local to World/state2FullState ==
  note: wrt GLOB
  note: Angles
      | wrtINI
  note: mode: Positioning
      | VelVEHICLE
      | wrt INI
  note: mode: Dynamics
      | VelVEHICLE
      | wrt VEH
  note: AnglesBODY
      | wrt GLOB
  note: AnglesVEHICLE
      | wrtGLOB
  note: AnglesBODY
      | wrtVEH
  dx,dy,dz [m/s] R,P,Y [rad] : Inport
  ini VEHpos wrt GLOB axis system [m] : Inport  Port=2
  iniBODY Angles wrt VEH axis system [deg] : Inport  Port=3
  iniVEH Angles wrt GLOB axis system [deg] : Inport  Port=4
  Degrees to Radians : simulink_extras/Transformations/Degrees to Radians
  Degrees to Radians1 : simulink_extras/Transformations/Degrees to Radians
  Demux1 : Demux  Outputs=[3 3 3]
  Demux2 : Demux  Outputs=[2 1]
  Demux3 : Demux  Outputs=2
  Mux : Mux  Inputs=[3 3]
  Sum : Sum  Inputs=|++
  Sum1 : Sum
  Sum2 : Sum
  Sum3 : Sum
  Terminator : Terminator
  Transformation_BODY2GLOBAL1 : Subsystem
  limit roll : Subsystem
  mux2 : Mux  Inputs=3
  mux3 : Mux  Inputs=3
  pitch_vehicle : Constant  Value=0
  roll_vehicle : Constant  Value=0
  yaw_body : Constant  Value=0
  State : Outport
  wires:
  Demux3/2 -> mux2/2  "pitch"
  ini VEHpos wrt GLOB axis system [m]/1 -> Sum3/2
  Degrees to Radians/1 -> Sum2/2, Transformation_BODY2GLOBAL1/2(angles_BODYwrtGLOB_[rad])
  Degrees to Radians1/1 -> Sum1/2
  Demux3/1 -> mux2/1  "roll"
  Demux1/3 -> Demux2/1
  Demux2/1 -> Demux3/1
  Demux2/2 -> mux3/3  "yaw"
  Sum3/1 -> Mux/1  "PosVEH wrt  GLOB"
  Transformation_BODY2GLOBAL1/1(POSvector_GLOBAL_[m]) -> Sum3/1
  Sum1/1 -> Sum/1
  Demux1/1 -> Transformation_BODY2GLOBAL1/1(POSvector_BODY_[m])
  dx,dy,dz [m/s] R,P,Y [rad]/1 -> Demux1/1
  Sum2/1 -> Sum/2
  mux3/1 -> Sum2/1
  yaw_body/1 -> mux2/3  "yaw"
  mux2/1 -> Sum1/1
  pitch_vehicle/1 -> mux3/2  "pitch"
  roll_vehicle/1 -> mux3/1  "roll"
  Sum/1 -> limit roll/1(RPY)
  iniBODY Angles wrt VEH axis system [deg]/1 -> Degrees to Radians1/1
  iniVEH Angles wrt GLOB axis system [deg]/1 -> Degrees to Radians/1
  Mux/1 -> State/1
  limit roll/1(RPYcor) -> Mux/2  "AnglesBODY wrt  GLOB"
  Demux1/2 -> Terminator/1

== system LMS_cs_old/BMW_X5_SUV_8/PreScan_Contact_Sensor/Wheels = 4/wheelposeFL ==
  vector : Inport  OutDataTypeStr=double  PortDimensions=7
  Bus Creator : BusCreator  Inputs='POSITION','ORIENTATION'  OutDataTypeStr=Bus: PRESCAN_POSEA_DATA  NonVirtualBus=on
  Bus Creator1 : BusCreator  Inputs='X','Y','Z'  OutDataTypeStr=Bus: PRESCAN_XYZ_DATA  NonVirtualBus=on
  Bus Creator3 : BusCreator  Inputs='X','Y','Z','Angle'  OutDataTypeStr=Bus: PRESCAN_AXISANGLE_DATA  NonVirtualBus=on
  Demux : Demux  Outputs=7
  bus : Outport  OutDataTypeStr=Bus: PRESCAN_POSEA_DATA
  wires:
  Bus Creator1/1 -> Bus Creator/1  "POSITION"
  Bus Creator3/1 -> Bus Creator/2  "ORIENTATION"
  Bus Creator/1 -> bus/1
  Demux/1 -> Bus Creator1/1  "X"
  Demux/2 -> Bus Creator1/2  "Y"
  Demux/3 -> Bus Creator1/3  "Z"
  Demux/4 -> Bus Creator3/1  "X"
  Demux/5 -> Bus Creator3/2  "Y"
  Demux/6 -> Bus Creator3/3  "Z"
  Demux/7 -> Bus Creator3/4  "Angle"
  vector/1 -> Demux/1

== system LMS_cs_old/BMW_X5_SUV_8/PreScan_Contact_Sensor/Wheels = 4/wheelposeFR ==
  vector : Inport  OutDataTypeStr=double  PortDimensions=7
  Bus Creator : BusCreator  Inputs='POSITION','ORIENTATION'  OutDataTypeStr=Bus: PRESCAN_POSEA_DATA  NonVirtualBus=on
  Bus Creator1 : BusCreator  Inputs='X','Y','Z'  OutDataTypeStr=Bus: PRESCAN_XYZ_DATA  NonVirtualBus=on
  Bus Creator3 : BusCreator  Inputs='X','Y','Z','Angle'  OutDataTypeStr=Bus: PRESCAN_AXISANGLE_DATA  NonVirtualBus=on
  Demux : Demux  Outputs=7
  bus : Outport  OutDataTypeStr=Bus: PRESCAN_POSEA_DATA
  wires:
  Bus Creator1/1 -> Bus Creator/1  "POSITION"
  Bus Creator3/1 -> Bus Creator/2  "ORIENTATION"
  Bus Creator/1 -> bus/1
  Demux/1 -> Bus Creator1/1  "X"
  Demux/2 -> Bus Creator1/2  "Y"
  Demux/3 -> Bus Creator1/3  "Z"
  Demux/4 -> Bus Creator3/1  "X"
  Demux/5 -> Bus Creator3/2  "Y"
  Demux/6 -> Bus Creator3/3  "Z"
  Demux/7 -> Bus Creator3/4  "Angle"
  vector/1 -> Demux/1

== system LMS_cs_old/BMW_X5_SUV_8/PreScan_Contact_Sensor/Wheels = 4/wheelposeRL ==
  vector : Inport  OutDataTypeStr=double  PortDimensions=7
  Bus Creator : BusCreator  Inputs='POSITION','ORIENTATION'  OutDataTypeStr=Bus: PRESCAN_POSEA_DATA  NonVirtualBus=on
  Bus Creator1 : BusCreator  Inputs='X','Y','Z'  OutDataTypeStr=Bus: PRESCAN_XYZ_DATA  NonVirtualBus=on
  Bus Creator3 : BusCreator  Inputs='X','Y','Z','Angle'  OutDataTypeStr=Bus: PRESCAN_AXISANGLE_DATA  NonVirtualBus=on
  Demux : Demux  Outputs=7
  bus : Outport  OutDataTypeStr=Bus: PRESCAN_POSEA_DATA
  wires:
  Bus Creator1/1 -> Bus Creator/1  "POSITION"
  Bus Creator3/1 -> Bus Creator/2  "ORIENTATION"
  Bus Creator/1 -> bus/1
  Demux/1 -> Bus Creator1/1  "X"
  Demux/2 -> Bus Creator1/2  "Y"
  Demux/3 -> Bus Creator1/3  "Z"
  Demux/4 -> Bus Creator3/1  "X"
  Demux/5 -> Bus Creator3/2  "Y"
  Demux/6 -> Bus Creator3/3  "Z"
  Demux/7 -> Bus Creator3/4  "Angle"
  vector/1 -> Demux/1

== system LMS_cs_old/BMW_X5_SUV_8/PreScan_Contact_Sensor/Wheels = 4/wheelposeRR ==
  vector : Inport  OutDataTypeStr=double  PortDimensions=7
  Bus Creator : BusCreator  Inputs='POSITION','ORIENTATION'  OutDataTypeStr=Bus: PRESCAN_POSEA_DATA  NonVirtualBus=on
  Bus Creator1 : BusCreator  Inputs='X','Y','Z'  OutDataTypeStr=Bus: PRESCAN_XYZ_DATA  NonVirtualBus=on
  Bus Creator3 : BusCreator  Inputs='X','Y','Z','Angle'  OutDataTypeStr=Bus: PRESCAN_AXISANGLE_DATA  NonVirtualBus=on
  Demux : Demux  Outputs=7
  bus : Outport  OutDataTypeStr=Bus: PRESCAN_POSEA_DATA
  wires:
  Bus Creator1/1 -> Bus Creator/1  "POSITION"
  Bus Creator3/1 -> Bus Creator/2  "ORIENTATION"
  Bus Creator/1 -> bus/1
  Demux/1 -> Bus Creator1/1  "X"
  Demux/2 -> Bus Creator1/2  "Y"
  Demux/3 -> Bus Creator1/3  "Z"
  Demux/4 -> Bus Creator3/1  "X"
  Demux/5 -> Bus Creator3/2  "Y"
  Demux/6 -> Bus Creator3/3  "Z"
  Demux/7 -> Bus Creator3/4  "Angle"
  vector/1 -> Demux/1

== system LMS_cs_old/BMW_X5_SUV_8/PreScan_Contact_Sensor/Wheels Local to World/conv_RotWheelFL ==
  BryantISO [deg] : Inport
  Fcn10 : Fcn  Expr=cos(u(1))*sin(u(3))+sin(u(1))*sin(u(2))*cos(u(3))
  Fcn11 : Fcn  Expr=sin(u(1))*sin(u(3))-cos(u(1))*sin(u(2))*cos(u(3))
  Fcn12 : Fcn  Expr=-cos(u(2))*sin(u(3))
  Fcn13 : Fcn  Expr=cos(u(1))*cos(u(3))-sin(u(1))*sin(u(2))*sin(u(3))
  Fcn14 : Fcn  Expr=sin(u(1))*cos(u(3))+cos(u(1))*sin(u(2))*sin(u(3))
  Fcn15 : Fcn  Expr=sin(u(2))
  Fcn16 : Fcn  Expr=-sin(u(1))*cos(u(2))
  Fcn17 : Fcn  Expr=cos(u(1))*cos(u(2))
  Fcn9 : Fcn  Expr=cos(u(2))*cos(u(3))
  Mux1 : Mux  Inputs=9
  RotMat2AxisAngle : Subsystem
  deg2rad : Gain  Gain=pi/180
  xyz 2 zxy : Selector  InputPortWidth=3  IndexOptions=Index vector (dialog)  Indices=[3 1 2]  OutputSizes=1
  zxy 2 xyz : Selector  InputPortWidth=4  IndexOptions=Index vector (dialog)  Indices=[2 3 1 4]  OutputSizes=1
  QuaternionVisu [rad] : Outport
  wires:
  zxy 2 xyz/1 -> QuaternionVisu [rad]/1
  xyz 2 zxy/1 -> deg2rad/1
  deg2rad/1 -> Fcn17/1, Fcn16/1, Fcn15/1, Fcn14/1, Fcn13/1, Fcn12/1, Fcn11/1, Fcn10/1, Fcn9/1
  BryantISO [deg]/1 -> xyz 2 zxy/1  "BryantAngles rotx roty rotz Visu"
  RotMat2AxisAngle/1(Angles_Visu) -> zxy 2 xyz/1
  Mux1/1 -> RotMat2AxisAngle/1(RotMat_Visu)  "RotationMatrix Visu"
  Fcn17/1 -> Mux1/9
  Fcn16/1 -> Mux1/8
  Fcn15/1 -> Mux1/7
  Fcn14/1 -> Mux1/6
  Fcn13/1 -> Mux1/5
  Fcn12/1 -> Mux1/4
  Fcn11/1 -> Mux1/3
  Fcn10/1 -> Mux1/2
  Fcn9/1 -> Mux1/1

== system LMS_cs_old/BMW_X5_SUV_8/PreScan_Contact_Sensor/Wheels Local to World/conv_RotWheelFR ==
  BryantISO [deg] : Inport
  Fcn10 : Fcn  Expr=cos(u(1))*sin(u(3))+sin(u(1))*sin(u(2))*cos(u(3))
  Fcn11 : Fcn  Expr=sin(u(1))*sin(u(3))-cos(u(1))*sin(u(2))*cos(u(3))
  Fcn12 : Fcn  Expr=-cos(u(2))*sin(u(3))
  Fcn13 : Fcn  Expr=cos(u(1))*cos(u(3))-sin(u(1))*sin(u(2))*sin(u(3))
  Fcn14 : Fcn  Expr=sin(u(1))*cos(u(3))+cos(u(1))*sin(u(2))*sin(u(3))
  Fcn15 : Fcn  Expr=sin(u(2))
  Fcn16 : Fcn  Expr=-sin(u(1))*cos(u(2))
  Fcn17 : Fcn  Expr=cos(u(1))*cos(u(2))
  Fcn9 : Fcn  Expr=cos(u(2))*cos(u(3))
  Mux1 : Mux  Inputs=9
  RotMat2AxisAngle : Subsystem
  deg2rad : Gain  Gain=pi/180
  xyz 2 zxy : Selector  InputPortWidth=3  IndexOptions=Index vector (dialog)  Indices=[3 1 2]  OutputSizes=1
  zxy 2 xyz : Selector  InputPortWidth=4  IndexOptions=Index vector (dialog)  Indices=[2 3 1 4]  OutputSizes=1
  QuaternionVisu [rad] : Outport
  wires:
  zxy 2 xyz/1 -> QuaternionVisu [rad]/1
  xyz 2 zxy/1 -> deg2rad/1
  deg2rad/1 -> Fcn17/1, Fcn16/1, Fcn15/1, Fcn14/1, Fcn13/1, Fcn12/1, Fcn11/1, Fcn10/1, Fcn9/1
  BryantISO [deg]/1 -> xyz 2 zxy/1  "BryantAngles rotx roty rotz Visu"
  RotMat2AxisAngle/1(Angles_Visu) -> zxy 2 xyz/1
  Mux1/1 -> RotMat2AxisAngle/1(RotMat_Visu)  "RotationMatrix Visu"
  Fcn17/1 -> Mux1/9
  Fcn16/1 -> Mux1/8
  Fcn15/1 -> Mux1/7
  Fcn14/1 -> Mux1/6
  Fcn13/1 -> Mux1/5
  Fcn12/1 -> Mux1/4
  Fcn11/1 -> Mux1/3
  Fcn10/1 -> Mux1/2
  Fcn9/1 -> Mux1/1

== system LMS_cs_old/BMW_X5_SUV_8/PreScan_Contact_Sensor/Wheels Local to World/conv_RotWheelRL ==
  BryantISO [deg] : Inport
  Fcn10 : Fcn  Expr=cos(u(1))*sin(u(3))+sin(u(1))*sin(u(2))*cos(u(3))
  Fcn11 : Fcn  Expr=sin(u(1))*sin(u(3))-cos(u(1))*sin(u(2))*cos(u(3))
  Fcn12 : Fcn  Expr=-cos(u(2))*sin(u(3))
  Fcn13 : Fcn  Expr=cos(u(1))*cos(u(3))-sin(u(1))*sin(u(2))*sin(u(3))
  Fcn14 : Fcn  Expr=sin(u(1))*cos(u(3))+cos(u(1))*sin(u(2))*sin(u(3))
  Fcn15 : Fcn  Expr=sin(u(2))
  Fcn16 : Fcn  Expr=-sin(u(1))*cos(u(2))
  Fcn17 : Fcn  Expr=cos(u(1))*cos(u(2))
  Fcn9 : Fcn  Expr=cos(u(2))*cos(u(3))
  Mux1 : Mux  Inputs=9
  RotMat2AxisAngle : Subsystem
  deg2rad : Gain  Gain=pi/180
  xyz 2 zxy : Selector  InputPortWidth=3  IndexOptions=Index vector (dialog)  Indices=[3 1 2]  OutputSizes=1
  zxy 2 xyz : Selector  InputPortWidth=4  IndexOptions=Index vector (dialog)  Indices=[2 3 1 4]  OutputSizes=1
  QuaternionVisu [rad] : Outport
  wires:
  zxy 2 xyz/1 -> QuaternionVisu [rad]/1
  xyz 2 zxy/1 -> deg2rad/1
  deg2rad/1 -> Fcn17/1, Fcn16/1, Fcn15/1, Fcn14/1, Fcn13/1, Fcn12/1, Fcn11/1, Fcn10/1, Fcn9/1
  BryantISO [deg]/1 -> xyz 2 zxy/1  "BryantAngles rotx roty rotz Visu"
  RotMat2AxisAngle/1(Angles_Visu) -> zxy 2 xyz/1
  Mux1/1 -> RotMat2AxisAngle/1(RotMat_Visu)  "RotationMatrix Visu"
  Fcn17/1 -> Mux1/9
  Fcn16/1 -> Mux1/8
  Fcn15/1 -> Mux1/7
  Fcn14/1 -> Mux1/6
  Fcn13/1 -> Mux1/5
  Fcn12/1 -> Mux1/4
  Fcn11/1 -> Mux1/3
  Fcn10/1 -> Mux1/2
  Fcn9/1 -> Mux1/1

== system LMS_cs_old/BMW_X5_SUV_8/PreScan_Contact_Sensor/Wheels Local to World/conv_RotWheelRR ==
  BryantISO [deg] : Inport
  Fcn10 : Fcn  Expr=cos(u(1))*sin(u(3))+sin(u(1))*sin(u(2))*cos(u(3))
  Fcn11 : Fcn  Expr=sin(u(1))*sin(u(3))-cos(u(1))*sin(u(2))*cos(u(3))
  Fcn12 : Fcn  Expr=-cos(u(2))*sin(u(3))
  Fcn13 : Fcn  Expr=cos(u(1))*cos(u(3))-sin(u(1))*sin(u(2))*sin(u(3))
  Fcn14 : Fcn  Expr=sin(u(1))*cos(u(3))+cos(u(1))*sin(u(2))*sin(u(3))
  Fcn15 : Fcn  Expr=sin(u(2))
  Fcn16 : Fcn  Expr=-sin(u(1))*cos(u(2))
  Fcn17 : Fcn  Expr=cos(u(1))*cos(u(2))
  Fcn9 : Fcn  Expr=cos(u(2))*cos(u(3))
  Mux1 : Mux  Inputs=9
  RotMat2AxisAngle : Subsystem
  deg2rad : Gain  Gain=pi/180
  xyz 2 zxy : Selector  InputPortWidth=3  IndexOptions=Index vector (dialog)  Indices=[3 1 2]  OutputSizes=1
  zxy 2 xyz : Selector  InputPortWidth=4  IndexOptions=Index vector (dialog)  Indices=[2 3 1 4]  OutputSizes=1
  QuaternionVisu [rad] : Outport
  wires:
  zxy 2 xyz/1 -> QuaternionVisu [rad]/1
  xyz 2 zxy/1 -> deg2rad/1
  deg2rad/1 -> Fcn17/1, Fcn16/1, Fcn15/1, Fcn14/1, Fcn13/1, Fcn12/1, Fcn11/1, Fcn10/1, Fcn9/1
  BryantISO [deg]/1 -> xyz 2 zxy/1  "BryantAngles rotx roty rotz Visu"
  RotMat2AxisAngle/1(Angles_Visu) -> zxy 2 xyz/1
  Mux1/1 -> RotMat2AxisAngle/1(RotMat_Visu)  "RotationMatrix Visu"
  Fcn17/1 -> Mux1/9
  Fcn16/1 -> Mux1/8
  Fcn15/1 -> Mux1/7
  Fcn14/1 -> Mux1/6
  Fcn13/1 -> Mux1/5
  Fcn12/1 -> Mux1/4
  Fcn11/1 -> Mux1/3
  Fcn10/1 -> Mux1/2
  Fcn9/1 -> Mux1/1

== system LMS_cs_old/BMW_X5_SUV_8/PreScan_Contact_Sensor/Wheels Local to World/conv_TransWheelFL ==
  transISO [m] : Inport
  Gain1 : Gain  Gain=Gain_xISO
  Gain2 : Gain  Gain=Gain_yISO
  Gain3 : Gain  Gain=Gain_zISO
  Mux2 : Mux  Inputs=3
  Sum : Sum  Inputs=|++
  pos_ini_Visu : Subsystem
  transISO2Visu : Subsystem
  transVisu [m] : Outport
  wires:
  Gain3/1 -> Mux2/3
  Gain2/1 -> Mux2/2
  Gain1/1 -> Mux2/1
  Sum/1 -> transVisu [m]/1
  pos_ini_Visu/1(pos_ini_Visu) -> Sum/2
  Mux2/1 -> Sum/1
  transISO [m]/1 -> transISO2Visu/1(transISO)
  transISO2Visu/1(trans_x_Visu) -> Gain1/1
  transISO2Visu/2(trans_y_Visu) -> Gain2/1
  transISO2Visu/3(trans_z_Visu) -> Gain3/1

== system LMS_cs_old/BMW_X5_SUV_8/PreScan_Contact_Sensor/Wheels Local to World/conv_TransWheelFR ==
  transISO [m] : Inport
  Gain1 : Gain  Gain=Gain_xISO
  Gain2 : Gain  Gain=Gain_yISO
  Gain3 : Gain  Gain=Gain_zISO
  Mux2 : Mux  Inputs=3
  Sum : Sum  Inputs=|++
  pos_ini_Visu : Subsystem
  transISO2Visu : Subsystem
  transVisu [m] : Outport
  wires:
  Gain3/1 -> Mux2/3
  Gain2/1 -> Mux2/2
  Gain1/1 -> Mux2/1
  Sum/1 -> transVisu [m]/1
  pos_ini_Visu/1(pos_ini_Visu) -> Sum/2
  Mux2/1 -> Sum/1
  transISO [m]/1 -> transISO2Visu/1(transISO)
  transISO2Visu/1(trans_x_Visu) -> Gain1/1
  transISO2Visu/2(trans_y_Visu) -> Gain2/1
  transISO2Visu/3(trans_z_Visu) -> Gain3/1

== system LMS_cs_old/BMW_X5_SUV_8/PreScan_Contact_Sensor/Wheels Local to World/conv_TransWheelRL ==
  transISO [m] : Inport
  Gain1 : Gain  Gain=Gain_xISO
  Gain2 : Gain  Gain=Gain_yISO
  Gain3 : Gain  Gain=Gain_zISO
  Mux2 : Mux  Inputs=3
  Sum : Sum  Inputs=|++
  pos_ini_Visu : Subsystem
  transISO2Visu : Subsystem
  transVisu [m] : Outport
  wires:
  Gain3/1 -> Mux2/3
  Gain2/1 -> Mux2/2
  Gain1/1 -> Mux2/1
  Sum/1 -> transVisu [m]/1
  pos_ini_Visu/1(pos_ini_Visu) -> Sum/2
  Mux2/1 -> Sum/1
  transISO2Visu/3(trans_z_Visu) -> Gain3/1
  transISO2Visu/2(trans_y_Visu) -> Gain2/1
  transISO [m]/1 -> transISO2Visu/1(transISO)
  transISO2Visu/1(trans_x_Visu) -> Gain1/1

== system LMS_cs_old/BMW_X5_SUV_8/PreScan_Contact_Sensor/Wheels Local to World/conv_TransWheelRR ==
  transISO [m] : Inport
  Gain1 : Gain  Gain=Gain_xISO
  Gain2 : Gain  Gain=Gain_yISO
  Gain3 : Gain  Gain=Gain_zISO
  Mux2 : Mux  Inputs=3
  Sum : Sum  Inputs=|++
  pos_ini_Visu : Subsystem
  transISO2Visu : Subsystem
  transVisu [m] : Outport
  wires:
  Gain3/1 -> Mux2/3
  Gain2/1 -> Mux2/2
  Gain1/1 -> Mux2/1
  Sum/1 -> transVisu [m]/1
  pos_ini_Visu/1(pos_ini_Visu) -> Sum/2
  Mux2/1 -> Sum/1
  transISO2Visu/3(trans_z_Visu) -> Gain3/1
  transISO2Visu/2(trans_y_Visu) -> Gain2/1
  transISO [m]/1 -> transISO2Visu/1(transISO)
  transISO2Visu/1(trans_x_Visu) -> Gain1/1

== system LMS_cs_old/BMW_X5_SUV_8/SELF_Demux/compas converter/cart2compas ==
  Angle [deg] : Inport
  Constant : Constant  Value=90
  Constant1 : Constant  Value=360
  Gain : Gain  Gain=1/360
  Gain1 : Gain  Gain=360
  Gain2 : Gain  Gain=-1
  Rounding Function : Rounding
  Sum : Sum  Inputs=|-+
  Sum1 : Sum  Inputs=-+|
  Sum2 : Sum  Inputs=++|
  heading [deg] : Outport
  wires:
  Gain/1 -> Rounding Function/1
  Rounding Function/1 -> Gain1/1
  Gain1/1 -> Sum/1
  Angle [deg]/1 -> Sum1/2
  Sum/1 -> Gain2/1
  Sum1/1 -> Gain/1, Sum/2
  Constant/1 -> Sum1/1
  Gain2/1 -> Sum2/2
  Constant1/1 -> Sum2/1
  Sum2/1 -> heading [deg]/1
